simulink model "A_tenue_altitude_pente_filtre_BdG"  (R2019b)
settings: Solver=VariableStepAuto  StartTime=0.0  StopTime=tsim  RelTol=1e-3
values from neighbouring files (symbols this model uses):
  A_AM = [0 0 0 0 0 0 ... (first row only)    [Code_conduite_vol.m]
  B_AM = [0;Zm;-Zm;mm;0;0]    [Code_conduite_vol.m]
  C_AM = eye(6)    [Code_conduite_vol.m]
  D_AM = zeros(6,1)    [Code_conduite_vol.m]
  K_gamma = 0.315    [Code_conduite_vol.m]
  Kn_BdG = Wn_BdG^2*num_BdG    [Code_conduite_vol.m]
  Kq = 0.0785    [Code_conduite_vol.m]
  Kz_gamma = 0.00167    [Code_conduite_vol.m]
  SW_BdG = 1    [Code_conduite_vol.m]
  SW_filtre = 1    [Code_conduite_vol.m]
  tau_filtre_q = mm/K    [Code_conduite_vol.m]
  z_c = 10    [Code_conduite_vol.m]
undefined symbols (not defined in the file or in its folder): den_BdG
settings Model: Creator=Alexa  LastModifiedBy=natha
settings DebuggingCC: SFMachineParentedDataDiag=error

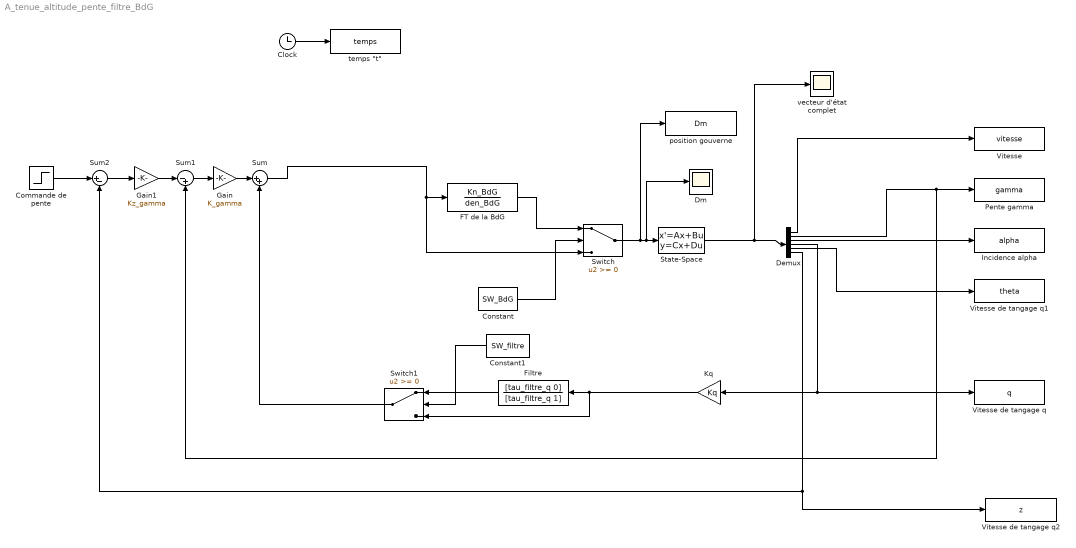
== system A_tenue_altitude_pente_filtre_BdG ==
  Clock : Clock
  Commande de pente : Step  Before=z_c  After=z_c  SampleTime=0
  Constant : Constant  Value=SW_BdG
  Constant1 : Constant  Value=SW_filtre
  Demux : Demux  Outputs=6
  Dm : Scope
  FT de la BdG : TransferFcn  Numerator=Kn_BdG  Denominator=den_BdG
  Filtre : TransferFcn  Numerator=[tau_filtre_q 0]  Denominator=[tau_filtre_q 1]
  Gain : Gain  Gain=K_gamma
  Gain1 : Gain  Gain=Kz_gamma
  Incidence alpha : ToWorkspace  VariableName=alpha  SampleTime=-1
  Kq : Gain  Gain=Kq
  Pente gamma : ToWorkspace  VariableName=gamma  SampleTime=-1
  State-Space : StateSpace  A=A_AM  B=B_AM  C=C_AM  D=D_AM  InitialCondition=0
  Sum : Sum  Inputs=|++
  Sum1 : Sum  Inputs=|-+
  Sum2 : Sum  Inputs=|+-
  Switch : Switch
  Switch1 : Switch
  Vitesse : ToWorkspace  VariableName=vitesse  SampleTime=-1
  Vitesse de tangage q : ToWorkspace  VariableName=q  SampleTime=-1
  Vitesse de tangage q1 : ToWorkspace  VariableName=theta  SampleTime=-1
  Vitesse de tangage q2 : ToWorkspace  VariableName=z  SampleTime=-1
  position gouverne : ToWorkspace  VariableName=Dm  SampleTime=-1
  "temps \"t\"" : ToWorkspace  VariableName=temps  SampleTime=-1
  "vecteur d'état complet " : Scope
  wires:
  Switch/1 -> position gouverne/1, Dm/1, State-Space/1
  FT de la BdG/1 -> Switch/1
  State-Space/1 -> Demux/1, "vecteur d'état complet "/1
  Constant/1 -> Switch/2
  Clock/1 -> "temps \"t\""/1
  Switch1/1 -> Sum/2
  Constant1/1 -> Switch1/2
  Filtre/1 -> Switch1/1
  Kq/1 -> Switch1/3, Filtre/1
  Demux/1 -> Vitesse/1
  Demux/2 -> Pente gamma/1, Sum1/2
  Demux/3 -> Incidence alpha/1
  Demux/4 -> Kq/1, Vitesse de tangage q/1
  Sum/1 -> Switch/3, FT de la BdG/1
  Sum1/1 -> Gain/1
  Gain/1 -> Sum/1
  Demux/5 -> Vitesse de tangage q1/1
  Demux/6 -> Sum2/2, Vitesse de tangage q2/1
  Commande de pente/1 -> Sum2/1
  Sum2/1 -> Gain1/1
  Gain1/1 -> Sum1/1
